simulink model "sampleModel2057"  (R2023a)
settings: Solver=VariableStepAuto  StartTime=0.0  StopTime=10.0  RelTol=1e-3
libraries: hdlsllib x5, simulink x1
settings Model: Creator=user1  LastModifiedBy=user1

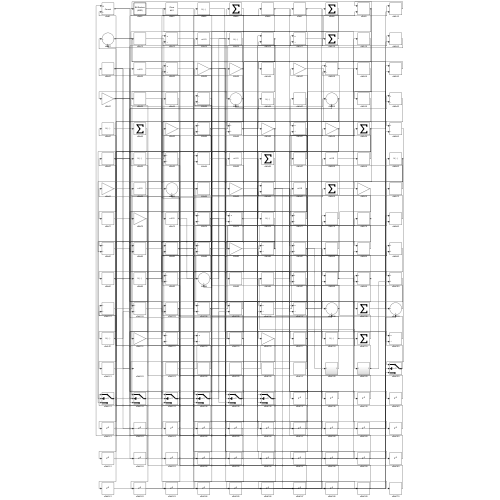
[thumbnail: Simulink's stored preview of the top-level diagram]
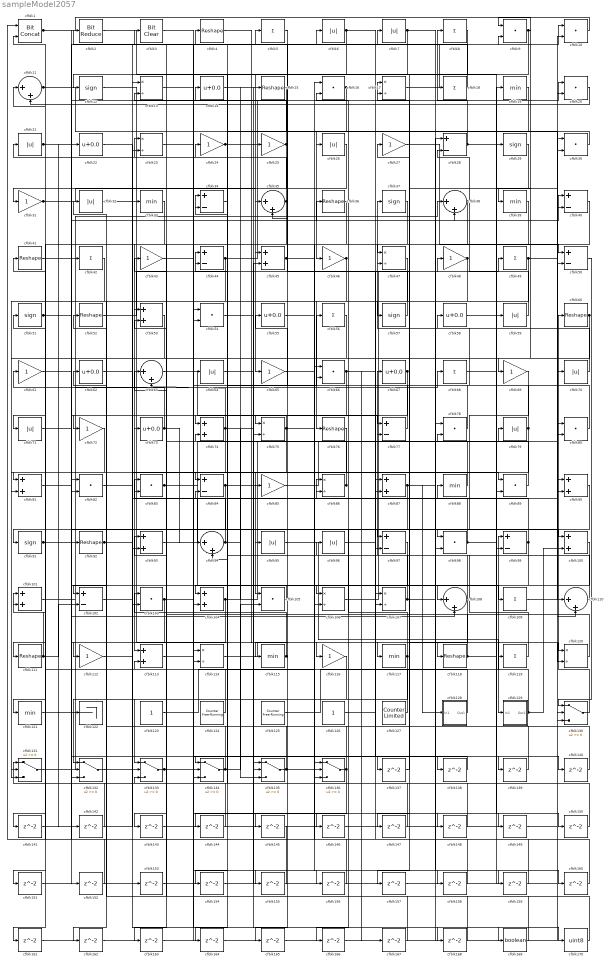
== system sampleModel2057 ==
  cfblk1 : hdlsllib/Logic and Bit Operations/Bit Concat  numInputs=2
  cfblk{9..10,16,20,30,54,66,78,80,82..83,89,98,103,105} (15 alike) : DotProduct  OutDataTypeStr=Inherit: Inherit via internal rule
  cfblk{45,53,74,81,87,90,93,100..101,104,113} (11 alike) : Sum
  cfblk{28,34,40,44,50,77,84,97,99,102} (10 alike) : Sum  Inputs=+-
  cfblk{13,17,23,47,75,86,106..107,114,120} (10 alike) : Product  Inputs=*/  RndMeth=Zero  SaturateOnIntegerOverflow=on
  cfblk{11,35,38,63,94,108,110} (7 alike) : Sum  Inputs=|++
  cfblk{5,8,18,42,49,56,68,109,119} (9 alike) : Sum  Inputs=+
  cfblk{4,15,36,41,52,60,76,92,111,118} (10 alike) : Reshape
  cfblk{24..25,27,31,43,46,48,61,65,69,72,85,112,116} (14 alike) : Gain
  cfblk{19,33,39,88,115,117,121} (7 alike) : MinMax
  cfblk{12,29,37,51,57,91} (6 alike) : Signum
  cfblk122 : Terminator
  cfblk123 : Constant  SampleTime=-1
  cfblk124 : hdlsllib/Sources/Counter Free-Running  NumBits=16  tsamp=-1
  cfblk125 : hdlsllib/Sources/Counter Free-Running  NumBits=16  tsamp=-1
  cfblk126 : Constant  SampleTime=-1
  cfblk127 : hdlsllib/Sources/Counter Limited  uplimit=7  tsamp=-1
  cfblk128 : Subsystem
      settings: LibrarySourceBlock=|
      | hdlsllib/Ports &
      | Subsystems/Subsystem
  cfblk129 : Subsystem
      settings: LibrarySourceBlock=|
      | hdlsllib/Ports &
      | Subsystems/Subsystem
  cfblk{130..136} (7 alike) : Switch  SaturateOnIntegerOverflow=off  InputSameDT=off
  cfblk{137..168} (32 alike) : Delay  SampleTime=1
  cfblk{14,22,55,58,62,67,73} (7 alike) : Bias  Bias=0.0  SaturateOnIntegerOverflow=off
  cfblk169 : DataTypeConversion  OutDataTypeStr=boolean  SaturateOnIntegerOverflow=off  RndMeth=Floor
  cfblk170 : DataTypeConversion  OutDataTypeStr=uint8  SaturateOnIntegerOverflow=off  RndMeth=Floor
  cfblk2 : hdlsllib/Logic and Bit Operations/Bit Reduce  mode=AND
  cfblk{6..7,21,26,32,59,64,70..71,79,95..96} (12 alike) : Abs  SaturateOnIntegerOverflow=off
  cfblk3 : simulink/Logic and Bit Operations/Bit Clear  iBit=0
      settings: LibrarySourceBlock=|
      | hdlsllib/Logic and Bit
      | Operations/Bit Clear
  wires:
  cfblk7/1 -> cfblk65/1, cfblk160/1
  cfblk106/1 -> cfblk49/1
  cfblk73/1 -> cfblk61/1, cfblk94/1
  cfblk4/1 -> cfblk116/1
  cfblk63/1 -> cfblk75/1
  cfblk1/1 -> cfblk69/1, cfblk103/2
  cfblk27/1 -> cfblk50/1
  cfblk24/1 -> cfblk135/1, cfblk149/1
  cfblk48/1 -> cfblk76/1, cfblk53/1
  cfblk37/1 -> cfblk113/1
  cfblk44/1 -> cfblk20/1, cfblk100/1, cfblk102/1
  cfblk104/1 -> cfblk60/1, cfblk132/3, cfblk15/1
  cfblk111/1 -> cfblk101/1, cfblk102/2
  cfblk115/1 -> cfblk131/1, cfblk53/2
  cfblk12/1 -> cfblk117/1
  cfblk112/1 -> cfblk88/1
  cfblk10/1 -> cfblk9/1
  cfblk95/1 -> cfblk129/1(In1)
  cfblk113/1 -> cfblk54/1
  cfblk46/1 -> cfblk131/2, cfblk151/1
  cfblk86/1 -> cfblk24/1, cfblk85/1, cfblk84/1
  cfblk131/1 -> cfblk68/1
  cfblk136/1 -> cfblk93/1, cfblk154/1
  cfblk34/1 -> cfblk134/1
  cfblk53/1 -> cfblk131/3
  cfblk28/1 -> cfblk8/1, cfblk40/2
  cfblk101/1 -> cfblk38/1
  cfblk17/1 -> cfblk9/2
  cfblk100/1 -> cfblk135/2
  cfblk36/1 -> cfblk73/1
  cfblk31/1 -> cfblk35/1, cfblk18/1, cfblk108/2
  cfblk70/1 -> cfblk37/1
  cfblk120/1 -> cfblk83/1
  cfblk47/1 -> cfblk111/1
  cfblk16/1 -> cfblk46/1, cfblk95/1
  cfblk78/1 -> cfblk55/1
  cfblk25/1 -> cfblk31/1, cfblk13/2
  cfblk89/1 -> cfblk23/1
  cfblk125/1 -> cfblk99/1
  cfblk77/1 -> cfblk56/1
  cfblk108/1 -> cfblk2/1, cfblk157/1
  cfblk8/1 -> cfblk47/1
  cfblk107/1 -> cfblk67/1, cfblk79/1, cfblk90/1
  cfblk135/1 -> cfblk52/1, cfblk148/1
  cfblk132/1 -> cfblk33/1
  cfblk94/1 -> cfblk43/1, cfblk25/1
  cfblk35/1 -> cfblk21/1, cfblk143/1
  cfblk85/1 -> cfblk30/1
  cfblk23/1 -> cfblk106/1
  cfblk99/1 -> cfblk14/1, cfblk115/1
  cfblk57/1 -> cfblk5/1
  cfblk38/1 -> cfblk57/1, cfblk137/1
  cfblk72/1 -> cfblk81/1
  cfblk133/1 -> cfblk10/1, cfblk146/1
  cfblk124/1 -> cfblk62/1
  cfblk60/1 -> cfblk162/1, cfblk163/1
  cfblk33/1 -> cfblk71/1
  cfblk5/1 -> cfblk45/1
  cfblk20/1 -> cfblk11/2
  cfblk129/1(Out1) -> cfblk119/1, cfblk100/2
  cfblk55/1 -> cfblk118/1
  cfblk118/1 -> cfblk59/1, cfblk74/2
  cfblk50/1 -> cfblk130/1
  cfblk116/1 -> cfblk132/1
  cfblk80/1 -> cfblk34/1
  cfblk88/1 -> cfblk17/1
  cfblk93/1 -> cfblk86/1
  cfblk83/1 -> cfblk78/2, cfblk136/3
  cfblk6/1 -> cfblk87/1, cfblk12/1
  cfblk61/1 -> cfblk7/1
  cfblk98/1 -> cfblk44/1, cfblk16/2, cfblk120/2
  cfblk62/1 -> cfblk13/1
  cfblk110/1 -> cfblk27/1
  cfblk82/1 -> cfblk89/1
  cfblk84/1 -> cfblk16/1, cfblk121/1
  cfblk105/1 -> cfblk104/1
  cfblk58/1 -> cfblk19/1
  cfblk127/1 -> cfblk41/1
  cfblk130/1 -> cfblk70/1
  cfblk92/1 -> cfblk6/1, cfblk84/2
  cfblk121/1 -> cfblk22/1
  cfblk2/1 -> cfblk99/2
  cfblk119/1 -> cfblk96/1
  cfblk18/1 -> cfblk4/1
  cfblk26/1 -> cfblk35/2
  cfblk51/1 -> cfblk38/2, cfblk108/1, cfblk97/2
  cfblk52/1 -> cfblk29/1
  cfblk75/1 -> cfblk40/1, cfblk72/1, cfblk112/1
  cfblk41/1 -> cfblk92/1
  cfblk13/1 -> cfblk64/1
  cfblk117/1 -> cfblk133/1, cfblk86/2
  cfblk11/1 -> cfblk110/1, cfblk104/2
  cfblk79/1 -> cfblk105/1, cfblk58/1
  cfblk123/1 -> cfblk106/2
  cfblk39/1 -> cfblk136/2
  cfblk67/1 -> cfblk74/1, cfblk75/2
  cfblk109/1 -> cfblk80/1
  cfblk114/1 -> cfblk120/1
  cfblk54/1 -> cfblk77/1
  cfblk128/1(Out1) -> cfblk51/1
  cfblk40/1 -> cfblk91/1
  cfblk21/1 -> cfblk42/1, cfblk122/1, cfblk142/1
  cfblk30/1 -> cfblk26/1
  cfblk59/1 -> cfblk28/2
  cfblk126/1 -> cfblk87/2
  cfblk45/1 -> cfblk109/1, cfblk17/2
  cfblk49/1 -> cfblk30/2, cfblk107/2, cfblk144/1
  cfblk69/1 -> cfblk98/1
  cfblk66/1 -> cfblk82/2, cfblk139/1, cfblk140/1, cfblk167/1
  cfblk91/1 -> cfblk133/2, cfblk36/1
  cfblk134/1 -> cfblk103/1, cfblk105/2
  cfblk56/1 -> cfblk114/2
  cfblk9/1 -> cfblk39/1, cfblk94/2
  cfblk32/1 -> cfblk97/1
  cfblk87/1 -> cfblk134/3, cfblk128/1(In1), cfblk90/2
  cfblk103/1 -> cfblk132/2, cfblk66/2
  cfblk96/1 -> cfblk48/1
  cfblk74/1 -> cfblk63/2, cfblk93/2, cfblk135/3, cfblk161/1, cfblk169/1
  cfblk76/1 -> cfblk81/2
  cfblk137/1 -> cfblk47/2
  cfblk71/1 -> cfblk138/1
  cfblk138/1 -> cfblk134/2
  cfblk139/1 -> cfblk77/2
  cfblk140/1 -> cfblk34/2
  cfblk42/1 -> cfblk141/1
  cfblk141/1 -> cfblk23/2
  cfblk142/1 -> cfblk101/2
  cfblk143/1 -> cfblk130/2
  cfblk144/1 -> cfblk83/2
  cfblk97/1 -> cfblk145/1
  cfblk145/1 -> cfblk1/1
  cfblk146/1 -> cfblk28/1
  cfblk29/1 -> cfblk147/1
  cfblk147/1 -> cfblk44/2
  cfblk148/1 -> cfblk1/2
  cfblk149/1 -> cfblk50/2
  cfblk68/1 -> cfblk150/1
  cfblk150/1 -> cfblk136/1
  cfblk151/1 -> cfblk80/2
  cfblk81/1 -> cfblk152/1
  cfblk152/1 -> cfblk82/1
  cfblk22/1 -> cfblk153/1
  cfblk153/1 -> cfblk45/2
  cfblk154/1 -> cfblk10/2
  cfblk43/1 -> cfblk155/1
  cfblk155/1 -> cfblk133/3
  cfblk14/1 -> cfblk156/1
  cfblk156/1 -> cfblk66/1
  cfblk157/1 -> cfblk89/2
  cfblk64/1 -> cfblk158/1
  cfblk158/1 -> cfblk63/1
  cfblk65/1 -> cfblk159/1
  cfblk159/1 -> cfblk11/1
  cfblk160/1 -> cfblk107/1
  cfblk161/1 -> cfblk130/3
  cfblk162/1 -> cfblk54/2
  cfblk163/1 -> cfblk98/2
  cfblk15/1 -> cfblk164/1
  cfblk164/1 -> cfblk110/2
  cfblk19/1 -> cfblk165/1
  cfblk165/1 -> cfblk20/2
  cfblk90/1 -> cfblk166/1
  cfblk166/1 -> cfblk78/1
  cfblk167/1 -> cfblk113/2
  cfblk102/1 -> cfblk168/1
  cfblk168/1 -> cfblk114/1
  cfblk169/1 -> cfblk3/1
  cfblk3/1 -> cfblk170/1
  cfblk170/1 -> cfblk32/1

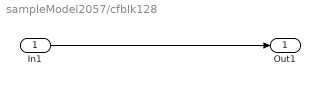
== system sampleModel2057/cfblk128 ==
  In1 : Inport
  Out1 : Outport
  wires:
  In1/1 -> Out1/1

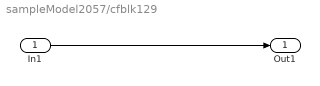
== system sampleModel2057/cfblk129 ==
  In1 : Inport
  Out1 : Outport
  wires:
  In1/1 -> Out1/1
